simulink model "shuangxiangquanqiao_DC"  (R2022b)
settings: Solver=ode23tb  StartTime=0.0  StopTime=1  MaxStep=0.02  RelTol=1e-4  EnableMultiTasking=on
libraries: spsIGBTDiodeLib x8, spsVoltageMeasurementLib x5, spsSeriesRLCBranchLib x4, spsCurrentMeasurementLib x3, spsLinearTransformerLib x1, sps_lib x1
Description:
  | Copyright 2008-2009 The MathWorks(TM), Inc.
settings Model: Creator=IREQ, Hydro-Quebec  LastModifiedBy=Loki
settings SolverCC: AlgebraicLoopSolver=TrustRegion
settings DataIOCC: LimitDataPoints=on  SaveFormat=Array  SignalLoggingSaveFormat=ModelDataLogs  ReturnWorkspaceOutputs=off
settings OptimizationCC: ExpressionDepthLimit=2147483647  InitFltsAndDblsToZero=on  LifeSpan=inf
settings DebuggingCC: SaveWithParameterizedLinksMsg=none  UnderspecifiedInitializationDetection=Classic  MergeDetectMultiDrivingBlocksExec=none  SignalResolutionControl=TryResolveAllWithWarning  SolverPrmCheckMsg=warning  MultiTaskDSMMsg=warning  MultiTaskCondExecSysMsg=none  FcnCallInpInsideContextMsg=warning  UnconnectedInputMsg=warning  UnconnectedOutputMsg=warning  UnconnectedLineMsg=warning  StateNameClashWarn=warning  SFUnexpectedBacktrackingDiag=warning  SFNoUnconditionalDefaultTransitionDiag=warning  SFExecutionAtInitializationDiag=none  SFMachineParentedDataDiag=warning  ArithmeticOperatorsInVariantConditions=warning
settings HardwareCC: ProdBitPerPointer=32  ProdBitPerSizeT=32  ProdBitPerPtrDiffT=32  ProdLargestAtomicFloat=None  ProdIntDivRoundTo=Undefined  ProdEndianess=Unspecified  ProdWordSize=32  ProdHWDeviceType=32-bit Generic
settings ModelReferenceCC: PropagateSignalLabelsOutOfModel=off
settings SFSimCC: SimUseLocalCustomCode=off  CustomCodeUndefinedFunction=UseInterfaceOnly
settings RTWCC: RTWUseLocalCustomCode=off
settings CodeAppCC: StateflowObjectComments=on
settings GRTTargetCC: TargetFcnLib=ansi_tfl_tmw.mat  TargetLangStandard=C89/C90 (ANSI)  CombineOutputUpdateFcns=off  GRTInterface=on
settings ConfigComp: CovMetricSettings=dw  CovSaveCumulativeToWorkspaceVar=on  CovSaveSingleToWorkspaceVar=on  CovExternalEMLEnable=off  CovSFcnEnable=off
settings SimscapeCC: SimscapeNormalizeSystem=off

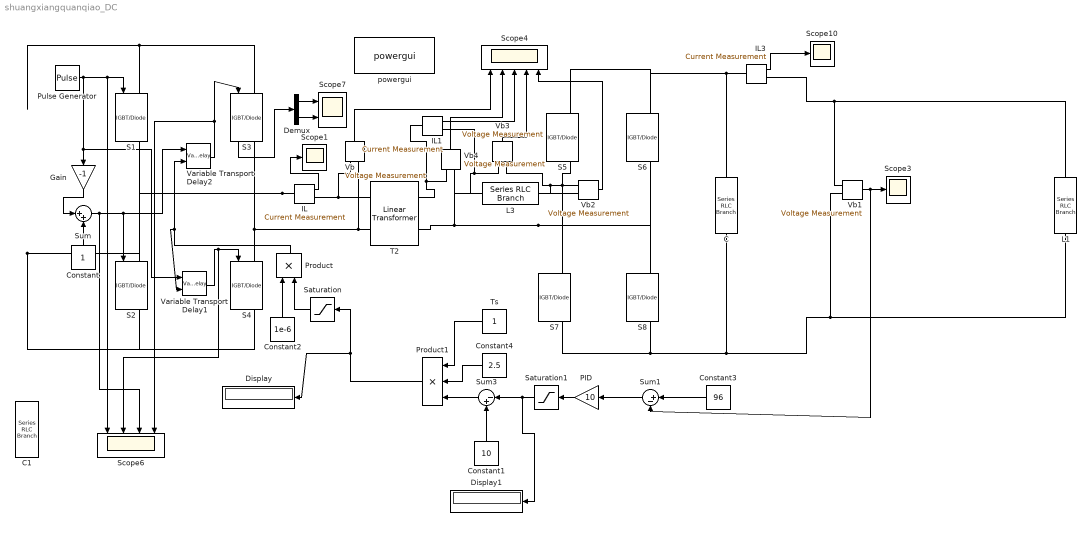
== system shuangxiangquanqiao_DC ==
  C : spsSeriesRLCBranchLib/Series RLC Branch  LConnTagsString=__new0  RConnTagsString=__new0  BranchType=C  Resistance=0.01  Inductance=1.0  SetiL0=on  InitialCurrent=0  Capacitance=1e-3  Setx0=on  InitialVoltage=0  Measurements=Branch voltage and current
  C1 : spsSeriesRLCBranchLib/Series RLC Branch  LConnTagsString=__new0  RConnTagsString=__new0  BranchType=C  Resistance=0.01  Inductance=1.0  SetiL0=on  InitialCurrent=0  Capacitance=100  Setx0=on  InitialVoltage=200  Measurements=Branch voltage and current
  Constant : Constant
  Constant1 : Constant  Value=10
  Constant2 : Constant  Value=1e-6
  Constant3 : Constant  Value=96
  Constant4 : Constant  Value=2.5
  Demux : Demux  Outputs=2
  Display : Display
  Display1 : Display
  Gain : Gain  Gain=-1
  IL : spsCurrentMeasurementLib/Current Measurement  PhasorSimulation=off  OutputType=Complex  PSBequivalent=0
  IL1 : spsCurrentMeasurementLib/Current Measurement  PhasorSimulation=off  OutputType=Complex  PSBequivalent=0
  IL3 : spsCurrentMeasurementLib/Current Measurement  PhasorSimulation=off  OutputType=Complex  PSBequivalent=0
  L1 : spsSeriesRLCBranchLib/Series RLC Branch  LConnTagsString=__new0  RConnTagsString=__new0  BranchType=R  Resistance=50  Inductance=1.0  SetiL0=on  InitialCurrent=0  Capacitance=1e-6  Setx0=off  InitialVoltage=0  Measurements=Branch voltage and current
  L3 : spsSeriesRLCBranchLib/Series RLC Branch  LConnTagsString=__new0  RConnTagsString=__new0  BranchType=L  Resistance=0.000000000000001  Inductance=1e-4  SetiL0=off  InitialCurrent=0  Capacitance=1e-6  Setx0=off  InitialVoltage=0  Measurements=Branch voltage and current
  PID : Gain  Gain=10
  Product : Product  RndMeth=Zero
  Product1 : Product  Inputs=3  RndMeth=Zero
  Pulse Generator : DiscretePulseGenerator  PulseType=Time based  Period=1e-4  PulseWidth=50
  S{1..8} (8 alike) : spsIGBTDiodeLib/IGBT//Diode  Ron=1e-3  Rs=1e5  Cs=inf  Measurements=on
  Saturation : Saturate  UpperLimit=50  LowerLimit=1
  Saturation1 : Saturate  UpperLimit=9  LowerLimit=-9  ZeroCross=off
  Scope1 : Scope
  Scope10 : Scope
  Scope3 : Scope
  Scope4 : Scope  NumInputPorts=5
  Scope6 : Scope  NumInputPorts=4
  Scope7 : Scope  NumInputPorts=2
  Sum : Sum  Inputs=|++
  Sum1 : Sum  Inputs=|+-
  Sum3 : Sum  Inputs=|-+
  T2 : spsLinearTransformerLib/Linear Transformer  UNITS=SI  NominalPower=[ 5000 60]  winding1=[200 0 1e-6]  winding2=[800 0 1e-6]  ThreeWindings=off  winding3=[3.15e+005 0.7938 0.084225]  RmLm=[1e9 inf]  Measurements=None  DataType=on
  Ts : Constant
  Variable Transport Delay1 : VariableTransportDelay  VariableDelayType=Variable transport delay  MaximumDelay=10
  Variable Transport Delay2 : VariableTransportDelay  VariableDelayType=Variable transport delay  MaximumDelay=10
  Vb{,1..4} (5 alike) : spsVoltageMeasurementLib/Voltage Measurement  PhasorSimulation=off  OutputType=Complex  PSBequivalent=0
  powergui : sps_lib/powergui  SimulationMode=Discrete  SampleTime=1e-5  frequency=60  Iterations=50  frequencyindice=0  Pbase=100e6  ErrMax=1e-4  UnitsV=kV  UnitsW=MW  buscounter=0  FunctionMessages=off  echomessages=off  EnableUseOfTLC=off  CurrentSourceSwitches=off  DisableSnubberDevices=off  DisableRonSwitches=off  DisableVfSwitches=off  DisplayEquations=off  AutomaticDiscreteSolvers=off  SolverType=Tustin/Backward Euler (TBE)  Interpol=off  ExternalGateDelay=off  methode=off  Ts=0  x0status=blocks  SPID=off  SwTol=0  HookPort=off  NonlinearTolerance=1e-4  nMaxIteration=100  ContinueOnMaxIteration=off  RestoreLinks=warning  ResistiveCurrentMeasurement=off  Frange=[0:2:500]  Ylog=off  Xlog=on  ShowGrid=off  save=off  variable=ZData  structure=0  ZoomFFT=on  StartTime=0.0  cycles=1  DisplayStyle=1  fundamental=60  FreqAxis=off  MaxFrequency=1000  frequencyindicesteady=1  RmsSteady=1  display=off
  wires:
  Vb1/1 -> Scope3/1, Sum1/2
  S3/1 -> Demux/1
  Demux/1 -> Scope7/1
  Demux/2 -> Scope7/2
  IL3/1 -> Scope10/1
  Pulse Generator/1 -> S1/1, Scope6/1, Variable Transport Delay1/1, Gain/1
  Variable Transport Delay2/1 -> S3/1, Scope6/4
  Variable Transport Delay1/1 -> S4/1, Scope6/2
  Constant/1 -> Sum/2
  Gain/1 -> Sum/1
  Sum/1 -> S2/1, Variable Transport Delay2/1, Scope6/3
  Constant2/1 -> Product/1
  Product/1 -> Variable Transport Delay2/2, Variable Transport Delay1/2
  Constant3/1 -> Sum1/1
  Saturation/1 -> Product/2
  Product1/1 -> Saturation/1, Display/1
  IL/1 -> Scope1/1
  Vb/1 -> Scope4/1
  Vb2/1 -> Scope4/5
  Vb3/1 -> Scope4/4
  IL1/1 -> Scope4/3
  Vb4/1 -> Scope4/2
  Saturation1/1 -> Sum3/1, Display1/1
  Constant1/1 -> Sum3/2
  Sum1/1 -> PID/1
  PID/1 -> Saturation1/1
  Sum3/1 -> Product1/3
  Constant4/1 -> Product1/2
  Ts/1 -> Product1/1
  connections:
  S3/LConn1 -- S1/LConn1
  T2/LConn2 -- S3/RConn1 -- S4/LConn1 -- Vb/LConn2
  S4/RConn1 -- S2/RConn1
  S6/RConn1 -- S8/LConn1 -- Vb2/LConn2 -- T2/RConn2 -- Vb4/LConn2
  S8/RConn1 -- L1/RConn1 -- Vb1/LConn2 -- C/RConn1 -- S7/RConn1
  IL/LConn1 -- S2/LConn1 -- S1/RConn1
  L1/LConn1 -- IL3/RConn1 -- Vb1/LConn1
  T2/LConn1 -- IL/RConn1 -- Vb/LConn1
  IL1/RConn1 -- Vb3/LConn1 -- L3/LConn1
  T2/RConn1 -- IL1/LConn1 -- Vb4/LConn1
  S5/LConn1 -- S6/LConn1 -- IL3/LConn1 -- C/LConn1
  Vb3/LConn2 -- L3/RConn1 -- Vb2/LConn1 -- S5/RConn1 -- S7/LConn1
